simulink model "CommSys_14_Bus"  (Simulink 8.0)
settings: Solver=ode45  StartTime=0.0  StopTime=2000  RelTol=1e-3
libraries: PiccSIM x17
settings Model: Creator=svenda  LastModifiedBy=svenda
settings DataIOCC: SignalLoggingSaveFormat=ModelDataLogs
settings DebuggingCC: FcnCallInpInsideContextMsg=EnableAllAsWarning

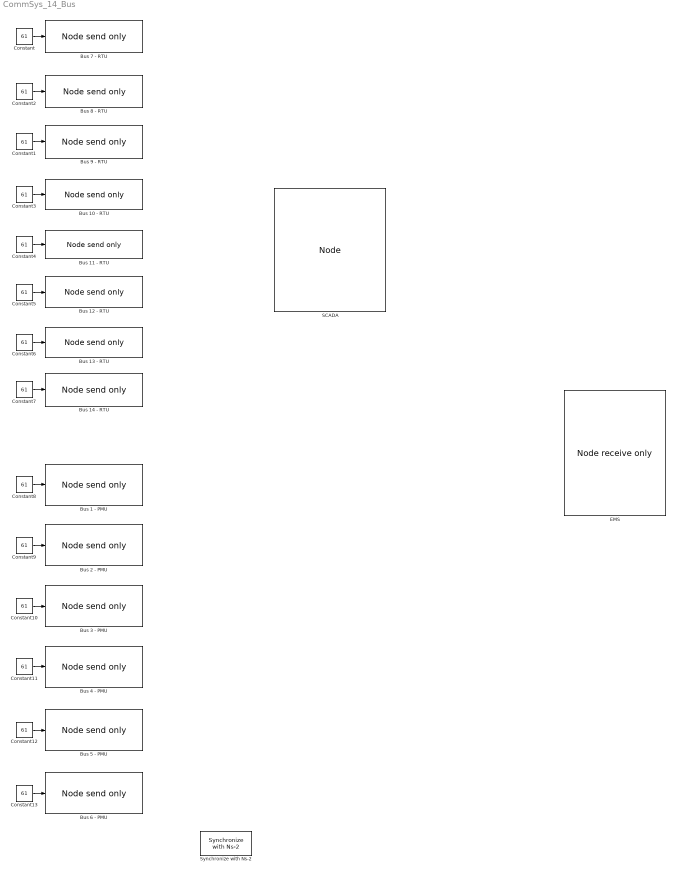
== system CommSys_14_Bus ==
  Bus 1 - PMU : PiccSIM/Node send only  ID=10  time_or_seq=Timestamp  sendSchedule=Fixed sampling time  h=0.02  duty_cycle=1  sendEnable=off  pTypesSend=[21]  sendDataStructure={{'double'}}  externalID=off  sendID={[9]}  coordinates=[0, 0]  IP=NS2_IP
  Bus 10 - RTU : PiccSIM/Node send only  ID=3  time_or_seq=Timestamp  sendSchedule=Fixed sampling time  h=2  duty_cycle=1  sendEnable=off  pTypesSend=[13]  sendDataStructure={{'double'}}  externalID=off  sendID={[8]}  coordinates=[0, 0]  IP=NS2_IP
  Bus 11 - RTU : PiccSIM/Node send only  ID=4  time_or_seq=Timestamp  sendSchedule=Fixed sampling time  h=2  duty_cycle=1  sendEnable=off  pTypesSend=[14]  sendDataStructure={{'double'}}  externalID=off  sendID={[8]}  coordinates=[0, 0]  IP=NS2_IP
  Bus 12 - RTU : PiccSIM/Node send only  ID=5  time_or_seq=Timestamp  sendSchedule=Fixed sampling time  h=2  duty_cycle=1  sendEnable=off  pTypesSend=[15]  sendDataStructure={{'double'}}  externalID=off  sendID={[8]}  coordinates=[0, 0]  IP=NS2_IP
  Bus 13 - RTU : PiccSIM/Node send only  ID=6  time_or_seq=Timestamp  sendSchedule=Fixed sampling time  h=2  duty_cycle=1  sendEnable=off  pTypesSend=[16]  sendDataStructure={{'double'}}  externalID=off  sendID={[8]}  coordinates=[0, 0]  IP=NS2_IP
  Bus 14 - RTU : PiccSIM/Node send only  ID=7  time_or_seq=Timestamp  sendSchedule=Fixed sampling time  h=2  duty_cycle=1  sendEnable=off  pTypesSend=[17]  sendDataStructure={{'double'}}  externalID=off  sendID={[8]}  coordinates=[0, 0]  IP=NS2_IP
  Bus 2 - PMU : PiccSIM/Node send only  ID=11  time_or_seq=Timestamp  sendSchedule=Fixed sampling time  h=0.02  duty_cycle=1  sendEnable=off  pTypesSend=[22]  sendDataStructure={{'double'}}  externalID=off  sendID={[9]}  coordinates=[0, 0]  IP=NS2_IP
  Bus 3 - PMU : PiccSIM/Node send only  ID=12  time_or_seq=Timestamp  sendSchedule=Fixed sampling time  h=0.02  duty_cycle=1  sendEnable=off  pTypesSend=[23]  sendDataStructure={{'double'}}  externalID=off  sendID={[9]}  coordinates=[0, 0]  IP=NS2_IP
  Bus 4 - PMU : PiccSIM/Node send only  ID=13  time_or_seq=Timestamp  sendSchedule=Fixed sampling time  h=0.02  duty_cycle=1  sendEnable=off  pTypesSend=[24]  sendDataStructure={{'double'}}  externalID=off  sendID={[9]}  coordinates=[0, 0]  IP=NS2_IP
  Bus 5 - PMU : PiccSIM/Node send only  ID=14  time_or_seq=Timestamp  sendSchedule=Fixed sampling time  h=0.02  duty_cycle=1  sendEnable=off  pTypesSend=[25]  sendDataStructure={{'double'}}  externalID=off  sendID={[9]}  coordinates=[0, 0]  IP=NS2_IP
  Bus 6 - PMU : PiccSIM/Node send only  ID=15  time_or_seq=Timestamp  sendSchedule=Fixed sampling time  h=0.02  duty_cycle=1  sendEnable=off  pTypesSend=[26]  sendDataStructure={{'double'}}  externalID=off  sendID={[9]}  coordinates=[0, 0]  IP=NS2_IP
  Bus 7 - RTU : PiccSIM/Node send only  ID=0  time_or_seq=Timestamp  sendSchedule=Fixed sampling time  h=2  duty_cycle=1  sendEnable=off  pTypesSend=[10]  sendDataStructure={{'double'}}  externalID=off  sendID={[8]}  coordinates=[0, 0]  IP=NS2_IP
  Bus 8 - RTU : PiccSIM/Node send only  ID=1  time_or_seq=Timestamp  sendSchedule=Fixed sampling time  h=2  duty_cycle=1  sendEnable=off  pTypesSend=[11]  sendDataStructure={{'double'}}  externalID=off  sendID={[8]}  coordinates=[0, 0]  IP=NS2_IP
  Bus 9 - RTU : PiccSIM/Node send only  ID=2  time_or_seq=Timestamp  sendSchedule=Fixed sampling time  h=2  duty_cycle=1  sendEnable=off  pTypesSend=[12]  sendDataStructure={{'double'}}  externalID=off  sendID={[8]}  coordinates=[0, 0]  IP=NS2_IP
  Constant{,1..13} (14 alike) : Constant  Value=61  OutDataTypeStr=double  SampleTime=1
  EMS : PiccSIM/Node receive only  ID=9  pTypes=[20,21,22,23,24,25,26]  receiveDataLengths={{[8]},{[1]},{[1]},{[1]},{[1]},{[1]},{[1]}}  receiveDataStructure={{'double'},{'double'},{'double'},{'double'},{'double'},{'double'},{'double'}}  recFrom={[8],[10],[11],[12],[13],[14],[15]}  coordinates=[0, 0]  IP=NS2_IP
  SCADA : PiccSIM/Node  ID=8  time_or_seq=Timestamp  sendSchedule=Fixed sampling time  h=2  duty_cycle=1  sendEnable=off  pTypesSend=[20]  sendDataStructure={{'double'}}  externalID=off  sendID={[9]}  pTypes=[10,11,12,13,14,15,16,17]  receiveDataLengths={{[1]},{[1]},{[1]},{[1]},{[1]},{[1]},{[1]},{[1]}}  receiveDataStructure={{'double'},{'double'},{'double'},{'double'},{'double'},{'double'},{'double'},{'double'}}  recFrom={[0],[1],[2],[3],[4],[5],[6],[7]}  coordinates=[1, 1]  IP=NS2_IP
  Synchronize with Ns-2 : PiccSIM/Synchronize with Ns-2  Priority=100000  c=1  port=23201  IP=NS2_IP
  wires:
  Constant/1 -> Bus 7 - RTU/1
  Constant2/1 -> Bus 8 - RTU/1
  Constant1/1 -> Bus 9 - RTU/1
  Constant3/1 -> Bus 10 - RTU/1
  Constant4/1 -> Bus 11 - RTU/1
  Constant5/1 -> Bus 12 - RTU/1
  Constant6/1 -> Bus 13 - RTU/1
  Constant7/1 -> Bus 14 - RTU/1
  Constant9/1 -> Bus 2 - PMU/1
  Constant10/1 -> Bus 3 - PMU/1
  Constant11/1 -> Bus 4 - PMU/1
  Constant12/1 -> Bus 5 - PMU/1
  Constant13/1 -> Bus 6 - PMU/1
  Constant8/1 -> Bus 1 - PMU/1
